simulink model "linearplant"  (R2015a)
settings: Solver=ode45  StartTime=0.0  StopTime=10.0  RelTol=1e-3
undefined symbols (not defined in the file or in its folder): A, B, C, D, K_lqr_toMotorcmd
settings Model: Creator=Sam  LastModifiedBy=Sam

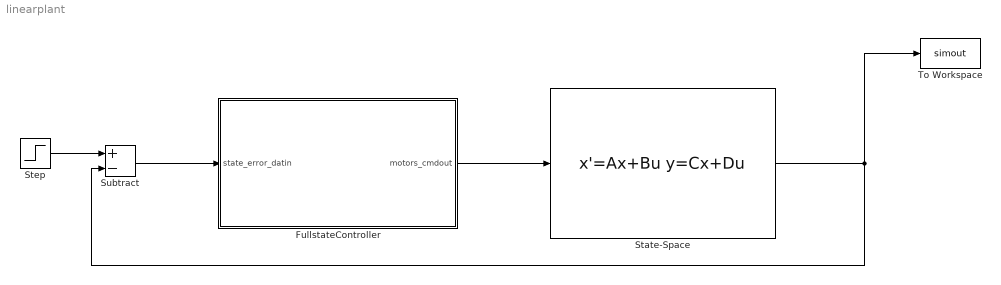
== system linearplant ==
  FullstateController : Subsystem
  State-Space : StateSpace  A=A  B=B  C=C  D=D  X0=[0;0;1.5;0;0;0;0;0;0;0;0;0]
  Step : Step  After=[0;0;-1.5;0;0;0;0;0;0;0;0;0]  SampleTime=0
  Subtract : Sum  Inputs=+-
  To Workspace : ToWorkspace  VariableName=simout  SaveFormat=Timeseries  SampleTime=-1
  wires:
  FullstateController/1(motors_cmdout) -> State-Space/1
  Subtract/1 -> FullstateController/1(state_error_datin)
  State-Space/1 -> To Workspace/1, Subtract/2
  Step/1 -> Subtract/1

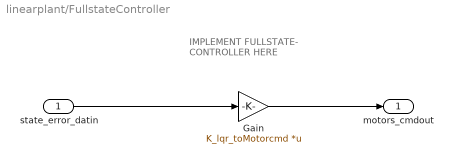
== system linearplant/FullstateController ==
  note: IMPLEMENT FULLSTATE-
      | CONTROLLER HERE
  state_error_datin : Inport
  Gain : Gain  Gain=K_lqr_toMotorcmd  Multiplication=Matrix(K*u)
  motors_cmdout : Outport
  wires:
  state_error_datin/1 -> Gain/1
  Gain/1 -> motors_cmdout/1
